simulink model "ricker_model"  (R2024b)
settings: Solver=VariableStepAuto  StartTime=0.0  StopTime=10.0  RelTol=1e-3
settings Model: Creator=Botló  LastModifiedBy=Botló

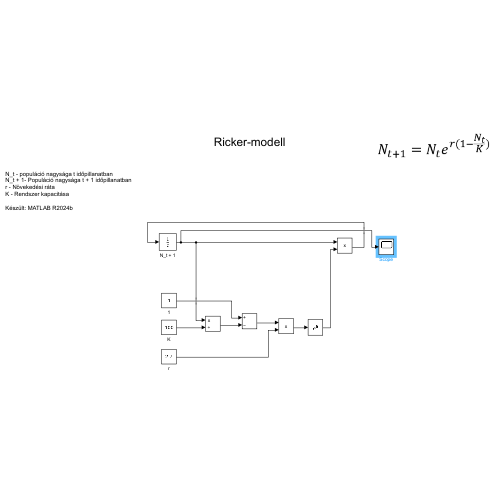
[thumbnail: Simulink's stored preview of the top-level diagram]
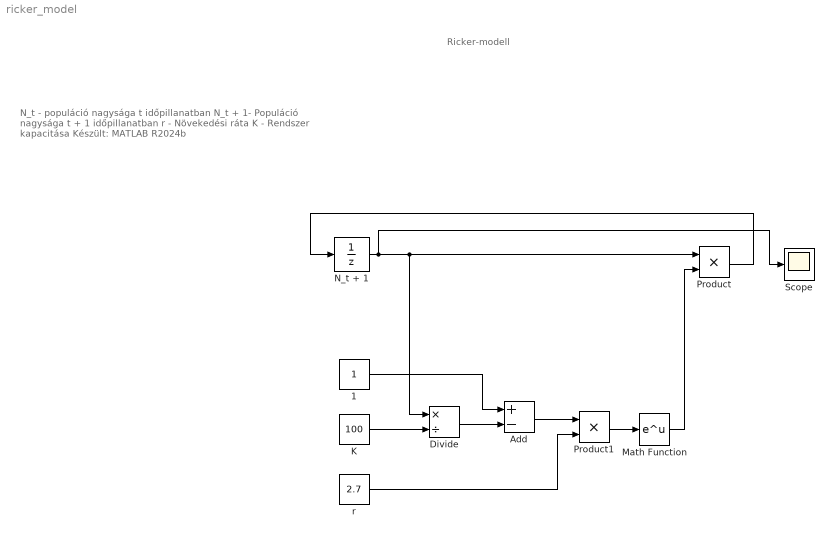
== system ricker_model ==
  note: Ricker-modell
  note: N_t - populáció nagysága t időpillanatban
      | N_t + 1- Populáció nagysága t + 1 időpillanatban
      | r - Növekedési ráta
      | K - Rendszer kapacitása
      |
      | Készült: MATLAB R2024b
  1 : Constant
  Add : Sum  Inputs=+-
  Divide : Product  Inputs=*/
  K : Constant  Value=100
  Math Function : Math
  N_t + 1 : UnitDelay  InitialCondition=10  SampleTime=-1  HasFrameUpgradeWarning=on
  Product : Product
  Product1 : Product
  Scope : Scope
  r : Constant  Value=2.7
  wires:
  K/1 -> Divide/2
  N_t + 1/1 -> Scope/1, Divide/1, Product/1
  Divide/1 -> Add/2
  1/1 -> Add/1
  Add/1 -> Product1/1
  r/1 -> Product1/2
  Product1/1 -> Math Function/1
  Math Function/1 -> Product/2
  Product/1 -> N_t + 1/1
